simulink model "model_podstawowy"  (R2020b)
settings: Solver=ode45  StartTime=0.0  StopTime=10  RelTol=1e-5
undefined symbols (not defined in the file): g, J, K_reg, L, M, m, th_konc, th_pocz
libraries: simulink x9
settings Model: Creator=maelstro  LastModifiedBy=maelstro
settings OptimizationCC: LifeSpan=inf
settings DebuggingCC: SFExecutionAtInitializationDiag=none  ArithmeticOperatorsInVariantConditions=warning
settings HardwareCC: ProdBitPerSizeT=32  ProdBitPerPtrDiffT=32  ProdWordSize=32  ProdHWDeviceType=Specified
settings SFSimCC: CustomCodeUndefinedFunction=UseInterfaceOnly
settings CodeAppCC: StateflowObjectComments=on

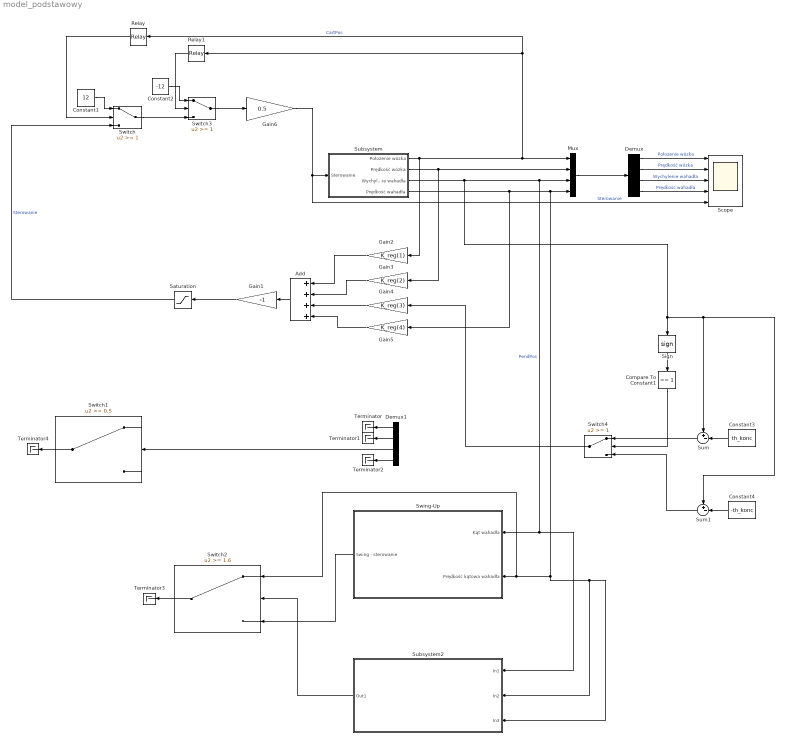
== system model_podstawowy ==
  Add : Sum  Inputs=++++
  Compare To Constant1 : simulink/Logic and Bit Operations/Compare To Constant  relop===  const=1  OutDataTypeStr=boolean
  Constant1 : Constant  Value=12
  Constant2 : Constant  Value=-12
  Constant3 : Constant  Value=th_konc
  Constant4 : Constant  Value=-th_konc
  Demux : Demux
  Demux1 : Demux
  Gain1 : Gain  Gain=-1
  Gain2 : Gain  Gain=K_reg(1)
  Gain3 : Gain  Gain=K_reg(2)
  Gain4 : Gain  Gain=K_reg(3)
  Gain5 : Gain  Gain=K_reg(4)
  Gain6 : Gain  Gain=0.5
  Mux : Mux
  Relay : Relay  OnSwitchValue=0.7  OffSwitchValue=0.6
  Relay1 : Relay  OnSwitchValue=-0.6  OffSwitchValue=-0.7  OnOutputValue=0  OffOutputValue=1
  Saturation : Saturate  UpperLimit=12  LowerLimit=-12
  Scope : Scope  NumInputPorts=5
  Sign : Signum
  Subsystem : Subsystem
  Subsystem2 : Subsystem
  Sum : Sum  Inputs=+-|
  Sum1 : Sum  Inputs=+-|
  Swing-Up : Subsystem
  Switch : Switch  Threshold=1
  Switch1 : Switch  Threshold=0.5
  Switch2 : Switch  Threshold=1.6
  Switch3 : Switch  Threshold=1
  Switch4 : Switch  Threshold=1
  Terminator{,1..4} (5 alike) : Terminator
  wires:
  Mux/1 -> Demux/1
  Subsystem/2(Prędkość wózka) -> Gain3/1, Mux/2
  Demux/1 -> Scope/1  "Położenie wózka"
  Demux/2 -> Scope/2  "Prędkość wózka"
  Demux/3 -> Scope/3  "Wychylenie wahadła"
  Demux/4 -> Scope/4  "Prędkość wahadła"
  Subsystem/4(Prędkość wahadła) -> Subsystem2/3(In3), Subsystem2/2(In2), Switch2/1, Swing-Up/2(Prędkość kątowa wahadła), Mux/4, Gain5/1
  Subsystem2/1(Out1) -> Switch2/2
  Swing-Up/1(Swing - sterowanie) -> Switch2/3
  Demux1/4 -> Terminator2/1
  Demux1/2 -> Terminator1/1
  Demux1/1 -> Terminator/1
  Demux1/3 -> Switch1/2
  Switch2/1 -> Terminator3/1
  Switch1/1 -> Terminator4/1
  Subsystem/1(Położenie wózka) -> Gain2/1, Relay/1, Relay1/1, Mux/1  "CartPos"
  Constant2/1 -> Switch3/1
  Relay/1 -> Switch/2
  Constant1/1 -> Switch/1
  Relay1/1 -> Switch3/2
  Saturation/1 -> Switch/3  "Sterowanie"
  Switch/1 -> Switch3/3
  Add/1 -> Gain1/1
  Switch4/1 -> Gain4/1
  Gain5/1 -> Add/4
  Gain4/1 -> Add/3
  Gain3/1 -> Add/2
  Gain2/1 -> Add/1
  Gain1/1 -> Saturation/1
  Switch3/1 -> Gain6/1
  Gain6/1 -> Scope/5, Subsystem/1(Sterowanie)  "Sterowanie"
  Subsystem/3(Wychylenie wahadła) -> Subsystem2/1(In1), Swing-Up/1(Kąt wahadła), Mux/3, Sum1/1, Sum/1, Sign/1  "PendPos"
  Constant3/1 -> Sum/2
  Sign/1 -> Compare To Constant1/1
  Sum/1 -> Switch4/1
  Constant4/1 -> Sum1/2
  Sum1/1 -> Switch4/3
  Compare To Constant1/1 -> Switch4/2

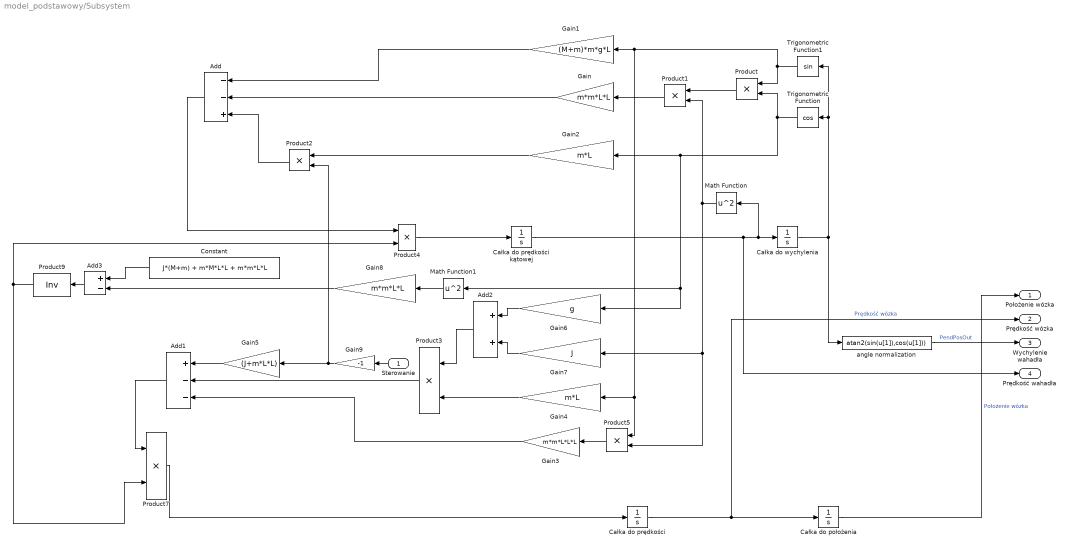
== system model_podstawowy/Subsystem ==
  Sterowanie : Inport
  Add : Sum  Inputs=--+
  Add1 : Sum  Inputs=+--
  Add2 : Sum
  Add3 : Sum  Inputs=+-
  Całka do położenia : Integrator
  Całka do prędkości : Integrator
  Całka do prędkości kątowej : Integrator
  Całka do wychylenia : Integrator  InitialCondition=th_pocz
  Constant : Constant  Value=J*(M+m) + m*M*L*L + m*m*L*L
  Gain : Gain  Gain=m*m*L*L
  Gain1 : Gain  Gain=(M+m)*m*g*L
  Gain2 : Gain  Gain=m*L
  Gain3 : Gain  Gain=m*m*L*L*L
  Gain4 : Gain  Gain=m*L
  Gain5 : Gain  Gain=(J+m*L*L)
  Gain6 : Gain  Gain=g
  Gain7 : Gain  Gain=J
  Gain8 : Gain  Gain=m*m*L*L
  Gain9 : Gain  Gain=-1
  Math Function : Math  Operator=square  SignedPower=on  SaturateOnIntegerOverflow=on
  Math Function1 : Math  Operator=square  SignedPower=on  SaturateOnIntegerOverflow=on
  Product{,1..5,7} (7 alike) : Product
  Product9 : Product  Inputs=/  Multiplication=Matrix(*)
  Trigonometric Function : Trigonometry  Operator=cos
  Trigonometric Function1 : Trigonometry
  angle normalization : Fcn  Expr=atan2(sin(u[1]),cos(u[1]))
  Położenie wózka : Outport
  Prędkość wózka : Outport  Port=2
  Wychylenie wahadła : Outport  Port=3
  Prędkość wahadła : Outport  Port=4
  wires:
  Add/1 -> Product4/1
  Całka do prędkości/1 -> Prędkość wózka/1, Całka do położenia/1  "Prędkość wózka"
  Gain4/1 -> Product3/2
  Product3/1 -> Add1/2
  Trigonometric Function/1 -> Math Function1/1, Gain6/1, Gain2/1, Product/2
  Gain2/1 -> Product2/1
  Product1/1 -> Gain/1
  Całka do położenia/1 -> Położenie wózka/1  "Położenie wózka"
  Trigonometric Function1/1 -> Product/1, Product5/1, Gain4/1, Gain1/1
  Product4/1 -> Całka do prędkości kątowej/1
  Gain/1 -> Add/2
  Gain1/1 -> Add/1
  Product/1 -> Product1/1
  Product2/1 -> Add/3
  Gain3/1 -> Add1/3
  Całka do prędkości kątowej/1 -> Prędkość wahadła/1, Math Function/1, Całka do wychylenia/1
  Gain5/1 -> Add1/1
  Math Function/1 -> Product1/2, Product5/2, Gain7/1
  Gain7/1 -> Add2/2
  Gain6/1 -> Add2/1
  Add2/1 -> Product3/1
  Product5/1 -> Gain3/1
  Add3/1 -> Product9/1
  Constant/1 -> Add3/1
  Gain8/1 -> Add3/2
  Math Function1/1 -> Gain8/1
  Product9/1 -> Product4/2, Product7/2
  Add1/1 -> Product7/1
  Product7/1 -> Całka do prędkości/1
  Całka do wychylenia/1 -> angle normalization/1, Trigonometric Function1/1, Trigonometric Function/1
  angle normalization/1 -> Wychylenie wahadła/1  "PendPosOut"
  Sterowanie/1 -> Gain9/1
  Gain9/1 -> Product2/2, Gain5/1

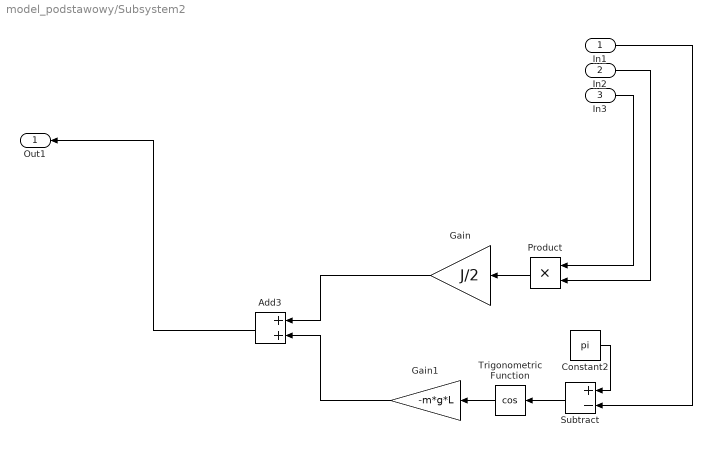
== system model_podstawowy/Subsystem2 ==
  In1 : Inport
  In2 : Inport  Port=2
  In3 : Inport  Port=3
  Add3 : Sum
  Constant2 : Constant  Value=pi
  Gain : Gain  Gain=J/2
  Gain1 : Gain  Gain=-m*g*L
  Product : Product
  Subtract : Sum  Inputs=+-
  Trigonometric Function : Trigonometry  Operator=cos
  Out1 : Outport
  wires:
  Trigonometric Function/1 -> Gain1/1
  Gain1/1 -> Add3/2
  Gain/1 -> Add3/1
  Constant2/1 -> Subtract/1
  Add3/1 -> Out1/1
  Product/1 -> Gain/1
  Subtract/1 -> Trigonometric Function/1
  In1/1 -> Subtract/2
  In2/1 -> Product/2
  In3/1 -> Product/1

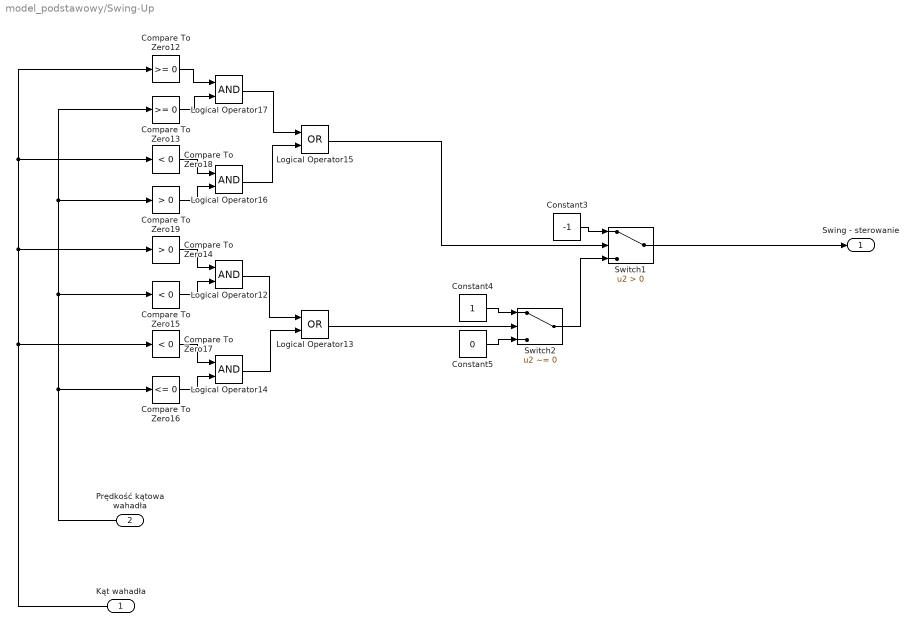
== system model_podstawowy/Swing-Up ==
  Kąt wahadła : Inport
  Prędkość kątowa wahadła : Inport  Port=2
  Compare To Zero12 : simulink/Logic and Bit Operations/Compare To Zero  relop=>=  OutDataTypeStr=uint8
  Compare To Zero13 : simulink/Logic and Bit Operations/Compare To Zero  relop=>=  OutDataTypeStr=uint8
  Compare To Zero14 : simulink/Logic and Bit Operations/Compare To Zero  relop=>  OutDataTypeStr=uint8
  Compare To Zero15 : simulink/Logic and Bit Operations/Compare To Zero  relop=<  OutDataTypeStr=uint8
  Compare To Zero16 : simulink/Logic and Bit Operations/Compare To Zero  relop=<=  OutDataTypeStr=uint8
  Compare To Zero17 : simulink/Logic and Bit Operations/Compare To Zero  relop=<  OutDataTypeStr=uint8
  Compare To Zero18 : simulink/Logic and Bit Operations/Compare To Zero  relop=<  OutDataTypeStr=uint8
  Compare To Zero19 : simulink/Logic and Bit Operations/Compare To Zero  relop=>  OutDataTypeStr=uint8
  Constant3 : Constant  Value=-1
  Constant4 : Constant
  Constant5 : Constant  Value=0
  Logical Operator{12,14,16..17} (4 alike) : Logic  AllPortsSameDT=off  OutDataTypeStr=boolean
  Logical Operator13 : Logic  Operator=OR  AllPortsSameDT=off  OutDataTypeStr=boolean
  Logical Operator15 : Logic  Operator=OR  AllPortsSameDT=off  OutDataTypeStr=boolean
  Switch1 : Switch  Criteria=u2 > Threshold
  Switch2 : Switch  Criteria=u2 ~= 0
  Swing - sterowanie : Outport
  wires:
  Prędkość kątowa wahadła/1 -> Compare To Zero15/1, Compare To Zero19/1, Compare To Zero13/1, Compare To Zero16/1
  Kąt wahadła/1 -> Compare To Zero17/1, Compare To Zero14/1, Compare To Zero18/1, Compare To Zero12/1
  Switch1/1 -> Swing - sterowanie/1
  Compare To Zero16/1 -> Logical Operator14/2
  Compare To Zero18/1 -> Logical Operator16/1
  Switch2/1 -> Switch1/3
  Logical Operator14/1 -> Logical Operator13/2
  Constant5/1 -> Switch2/3
  Logical Operator12/1 -> Logical Operator13/1
  Compare To Zero17/1 -> Logical Operator14/1
  Compare To Zero12/1 -> Logical Operator17/1
  Logical Operator16/1 -> Logical Operator15/2
  Compare To Zero14/1 -> Logical Operator12/1
  Constant4/1 -> Switch2/1
  Compare To Zero15/1 -> Logical Operator12/2
  Compare To Zero13/1 -> Logical Operator17/2
  Logical Operator17/1 -> Logical Operator15/1
  Logical Operator15/1 -> Switch1/2
  Constant3/1 -> Switch1/1
  Compare To Zero19/1 -> Logical Operator16/2
  Logical Operator13/1 -> Switch2/2
